simulink model "SL7_2_7"  (R2015b)
settings: Solver=VariableStepAuto  StartTime=0.0  StopTime=50.0  RelTol=1e-3
settings Model: Creator=Administrator  LastModifiedBy=Administrator

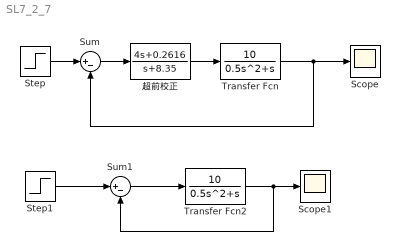
== system SL7_2_7 ==
  Scope : Scope
  Scope1 : Scope
  Step : Step  Time=0  SampleTime=0
  Step1 : Step  Time=0  SampleTime=0
  Sum : Sum  Inputs=|+-
  Sum1 : Sum  Inputs=|+-
  Transfer Fcn : TransferFcn  Numerator=[10]  Denominator=[0.5 1 0]
  Transfer Fcn2 : TransferFcn  Numerator=[10]  Denominator=[0.5 1 0]
  超前校正 : TransferFcn  Numerator=[4 0.2616]  Denominator=[1 8.35]
  wires:
  Transfer Fcn/1 -> Sum/2, Scope/1
  Step/1 -> Sum/1
  超前校正/1 -> Transfer Fcn/1
  Sum/1 -> 超前校正/1
  Transfer Fcn2/1 -> Sum1/2, Scope1/1
  Sum1/1 -> Transfer Fcn2/1
  Step1/1 -> Sum1/1
